simulink model "GbxNPos_DD"  (R2016b)
settings: configuration reference "CodeGenConfigSet" (kept outside this file)
values from neighbouring files (symbols this model uses):
  Gbx_NPosDeb_tiHiLo_C = Calibration.Parameter    [init_GbxNPos_DD.m]    (also in init_GbxNPos_DD_SIL.m = Simulink.Parameter)
  Gbx_NPosDeb_tiLoHi_C = Calibration.Parameter    [init_GbxNPos_DD.m]    (also in init_GbxNPos_DD_SIL.m = Simulink.Parameter)
undefined symbols (not defined in the file or in its folder): GbxNPos_DD_DT
libraries: CXLib x1
settings Model: Creator=bianxuyin  LastModifiedBy=bianxuyin
settings ConfigSetRef: SourceLocation=Base Workspace

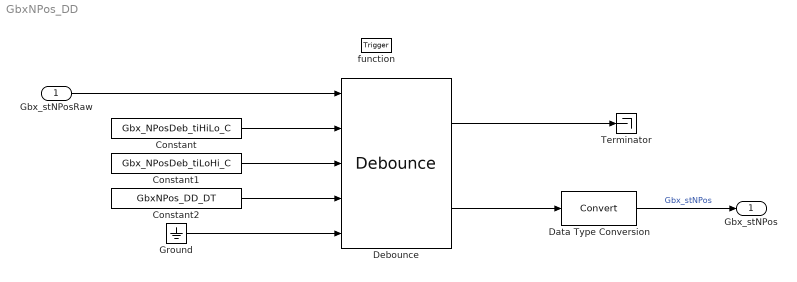
== system GbxNPos_DD ==
  Gbx_stNPosRaw : Inport  Description=Raw signal from the digital gearbox neutural position sensior  OutMin=0  OutMax=255  OutDataTypeStr=State_uint8
  function : TriggerPort  TriggerType=function-call  VariantControl=Variant
  Constant : Constant  Value=Gbx_NPosDeb_tiHiLo_C
  Constant1 : Constant  Value=Gbx_NPosDeb_tiLoHi_C
  Constant2 : Constant  Value=GbxNPos_DD_DT
  Data Type Conversion : DataTypeConversion
  Debounce : CXLib/Debounce
  Ground : Ground
  Terminator : Terminator
  Gbx_stNPos : Outport  Description=Gearbox neutral position status signal  OutMin=0  OutMax=255  OutDataTypeStr=State_uint8
  wires:
  Debounce/2 -> Data Type Conversion/1
  Gbx_stNPosRaw/1 -> Debounce/1
  Constant/1 -> Debounce/2
  Constant1/1 -> Debounce/3
  Constant2/1 -> Debounce/4
  Ground/1 -> Debounce/5
  Debounce/1 -> Terminator/1
  Data Type Conversion/1 -> Gbx_stNPos/1  "Gbx_stNPos"
